simulink model "Copy_1_of_sistema"  (R2025b)
settings: Solver=ode23t  StartTime=0.0  StopTime=10.0  MaxStep=1e-3  RelTol=1e-3
settings DataIOCC: ReturnWorkspaceOutputs=off  TimeSaveName=t
settings DebuggingCC: AlgebraicLoopMsg=none  ArtificialAlgebraicLoopMsg=none  MaxConsecutiveZCsMsg=none

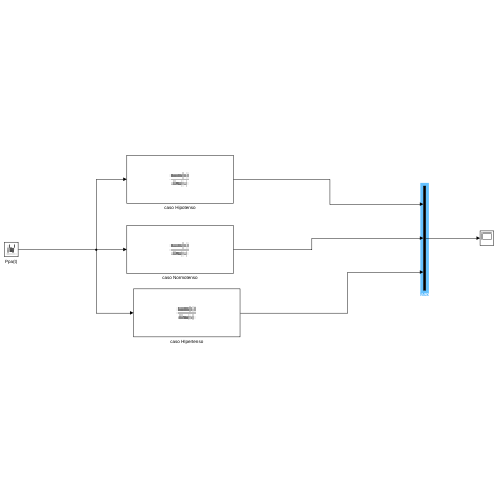
[thumbnail: Simulink's stored preview of the top-level diagram]
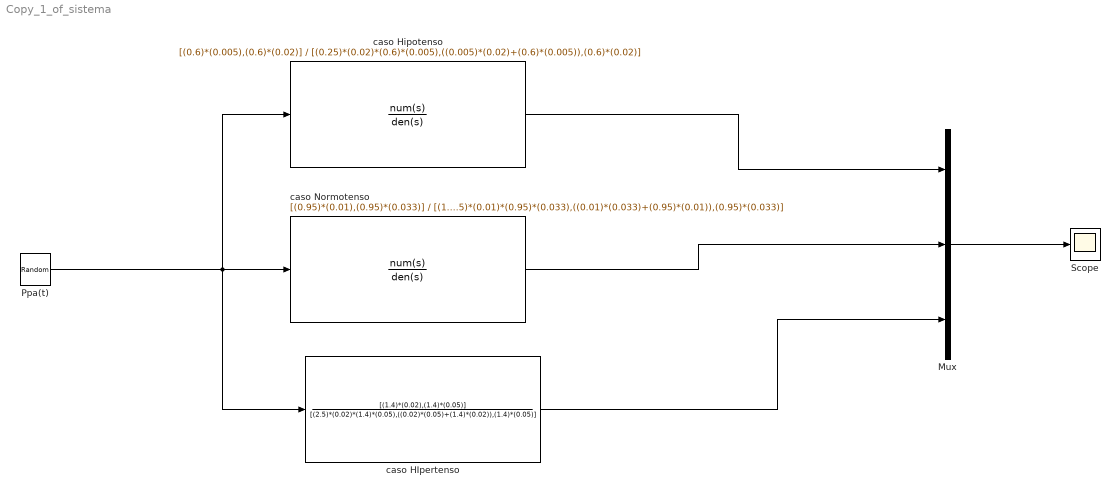
== system Copy_1_of_sistema ==
  Mux : Mux  Inputs=3
  Ppa(t) : UniformRandomNumber  Minimum=-0.2  Seed=106  SampleTime=0.5
  Scope : Scope
      settings: ActiveDisplayYMinimum=-0.85739249599732059  ActiveDisplayYMaximum=1.3241777304666695
  caso HIpertenso : TransferFcn  Numerator=[(1.4)*(0.02),(1.4)*(0.05)]  Denominator=[(2.5)*(0.02)*(1.4)*(0.05),((0.02)*(0.05)+(1.4)*(0.02)),(1.4)*(0.05)]
  caso Hipotenso : TransferFcn  Numerator=[(0.6)*(0.005),(0.6)*(0.02)]  Denominator=[(0.25)*(0.02)*(0.6)*(0.005),((0.005)*(0.02)+(0.6)*(0.005)),(0.6)*(0.02)]
  caso Normotenso : TransferFcn  Numerator=[(0.95)*(0.01),(0.95)*(0.033)]  Denominator=[(1.5)*(0.01)*(0.95)*(0.033),((0.01)*(0.033)+(0.95)*(0.01)),(0.95)*(0.033)]
  wires:
  Mux/1 -> Scope/1
  Ppa(t)/1 -> caso HIpertenso/1, caso Hipotenso/1, caso Normotenso/1
  caso HIpertenso/1 -> Mux/3
  caso Normotenso/1 -> Mux/2
  caso Hipotenso/1 -> Mux/1
